simulink model "FiveStateAbsTcs"  (R2023b)
settings: configuration reference "VehicleFixed1ms" (kept outside this file)
undefined symbols (not defined in the file): CtrlBcuTrlrBrkGain, DiscIntNeverNeededParam, PlntWhlLdRadius
libraries: simulink x2
settings Model: DataDictionary=VirtualVehicleTemplate.sldd  ModifiedByFormat=The MathWorks, Inc.  Creator=The MathWorks, Inc.  LastModifiedBy=The MathWorks, Inc.
settings ConfigSetRef: SourceName=VehicleFixed1ms

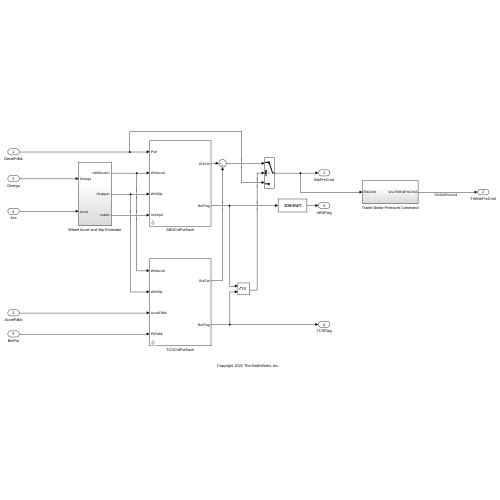
[thumbnail: Simulink's stored preview of the top-level diagram]
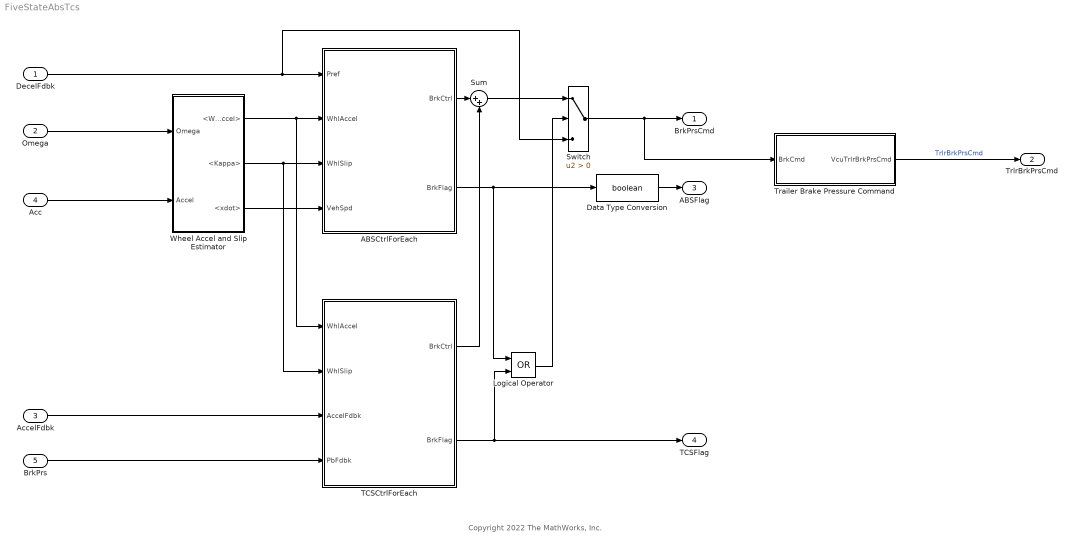
== system FiveStateAbsTcs ==
  note: Copyright 2022 The MathWorks, Inc.
  DecelFdbk : Inport  OutDataTypeStr=double  PortDimensions=1
  Omega : Inport  Port=2  OutDataTypeStr=double  PortDimensions=4
  AccelFdbk : Inport  Port=3  OutDataTypeStr=double  PortDimensions=1
  Acc : Inport  Port=4  OutDataTypeStr=double  PortDimensions=1
  BrkPrs : Inport  Port=5  OutDataTypeStr=double  PortDimensions=4
  ABSCtrlForEach : Subsystem  mask(Five-State ABS Control){Re=PlntWhlLdRadius, KappaOpt=-0.12, WhlAccelOpt=[-9.8,-9.8,-20,-20], v1=0, v5=0.55, v4=1, a2=-1.5, b=-1.5, A=4.5, a1=3.6, aMode=2}
      mask prompts: Re "Wheel effective radius, Re [m]:"; KappaOpt "Desired wheel slip ratio, KappaOpt [-]:"; WhlAccelOpt "Desired wheel acceleration, WhlAccelOpt [m/s^2]:"; v1 "Braking realease command, v1 [-]:"; v5 "Braking hold command, v5 [-]:"; v4 "Braking add command, v4 [-]:"; a2 "Threshold of State 1, a2 [m/s^2]:"; b "Threshold of State 2, b [m/s^2]:"; A "Threshold of State 3 and 4, A [m/s^2]:"; a1 "Threshold of State 5, a1 [m/s^2]:"
      mask help: This block determines brake pressure varying rate for each wheel once the ABS controller is activated. During ABS control, only wheel speed is directly regulated.
      mask init:
      | [~]=vehdynicon('vehdynblk',gcb);
      mask DialogControl vehParamGroup Prompt: Vehicle Parameter
      mask DialogControl ParameterGroupVar Prompt: Desired Control Parameters
      mask DialogControl Container3 Prompt: Braking Pressure Rates
      mask DialogControl Container4 Prompt: Wheel Acceleration Thresholds
  Data Type Conversion : DataTypeConversion  OutDataTypeStr=boolean  SaturateOnIntegerOverflow=off  RndMeth=Floor
  Logical Operator : Logic  Operator=OR  AllPortsSameDT=off  OutDataTypeStr=boolean
  Sum : Sum  Inputs=|++
  Switch : Switch  Criteria=u2 > Threshold  SaturateOnIntegerOverflow=off  InputSameDT=off
  TCSCtrlForEach : Subsystem  mask(Five-State TCS Control){Re=PlntWhlLdRadius, KappaOpt=0.12, WhlAccelOpt=[11, 11, 11, 11], v1=1.5, v5=-0.5, v4=-1.2, a2=-6, b=-10, A=-11, a1=-9, aMode=2}
      mask prompts: Re "Wheel effective radius, Re [m]:"; KappaOpt "Desired wheel slip ratio, KappaOpt [-]:"; WhlAccelOpt "Desired wheel acceleration, WhlAccelOpt [m/s^2]:"; v1 "Braking pressure rising rate, v1 [-]:"; v5 "Secondary braking pressure declining rate, v5 [-]:"; v4 "Braking pressure declining rate, v4 [-]:"; a2 "Threshold of State 1, a2 [m/s^2]:"; b "Threshold of State 2, b [m/s^2]:"; A "Threshold of State 3 and 4, A [m/s^2]:"; a1 "Threshold of State 5, a1 [m/s^2]:"
      mask help: This block determines brake pressure varying rate for each wheel once the TCS controller is activated. During TCS control, only wheel speed is directly regulated.
      mask init:
      | [~]=vehdynicon('vehdynblk',gcb);
      mask DialogControl vehParamGroup Prompt: Vehicle Parameter
      mask DialogControl ParameterGroupVar Prompt: Desired Control Parameters
      mask DialogControl Container3 Prompt: Braking Pressure Rates
      mask DialogControl Container4 Prompt: Wheel Acceleration Thresholds
  Trailer Brake Pressure Command : Subsystem
  Wheel Accel and Slip Estimator : Subsystem
  BrkPrsCmd : Outport  OutDataTypeStr=double  PortDimensions=4
  TrlrBrkPrsCmd : Outport  Port=2  PortDimensions=6  VectorParamsAs1DForOutWhenUnconnected=off
  ABSFlag : Outport  Port=3  OutDataTypeStr=boolean  PortDimensions=4
  TCSFlag : Outport  Port=4  OutDataTypeStr=double  PortDimensions=4
  wires:
  DecelFdbk/1 -> Switch/3, ABSCtrlForEach/1(Pref)
  Wheel Accel and Slip Estimator/3(<xdot>) -> ABSCtrlForEach/4(VehSpd)
  ABSCtrlForEach/1(BrkCtrl) -> Sum/1
  Sum/1 -> Switch/1
  BrkPrs/1 -> TCSCtrlForEach/4(PbFdbk)
  TCSCtrlForEach/1(BrkCtrl) -> Sum/2
  Logical Operator/1 -> Switch/2
  AccelFdbk/1 -> TCSCtrlForEach/3(AccelFdbk)
  Wheel Accel and Slip Estimator/1(<WhlAccel>) -> TCSCtrlForEach/1(WhlAccel), ABSCtrlForEach/2(WhlAccel)
  TCSCtrlForEach/2(BrkFlag) -> TCSFlag/1, Logical Operator/2
  ABSCtrlForEach/2(BrkFlag) -> Data Type Conversion/1, Logical Operator/1
  Wheel Accel and Slip Estimator/2(<Kappa>) -> TCSCtrlForEach/2(WhlSlip), ABSCtrlForEach/3(WhlSlip)
  Switch/1 -> Trailer Brake Pressure Command/1(BrkCmd), BrkPrsCmd/1
  Omega/1 -> Wheel Accel and Slip Estimator/1(Omega)
  Acc/1 -> Wheel Accel and Slip Estimator/2(Accel)
  Data Type Conversion/1 -> ABSFlag/1
  Trailer Brake Pressure Command/1(VcuTrlrBrkPrsCmd) -> TrlrBrkPrsCmd/1  "TrlrBrkPrsCmd"

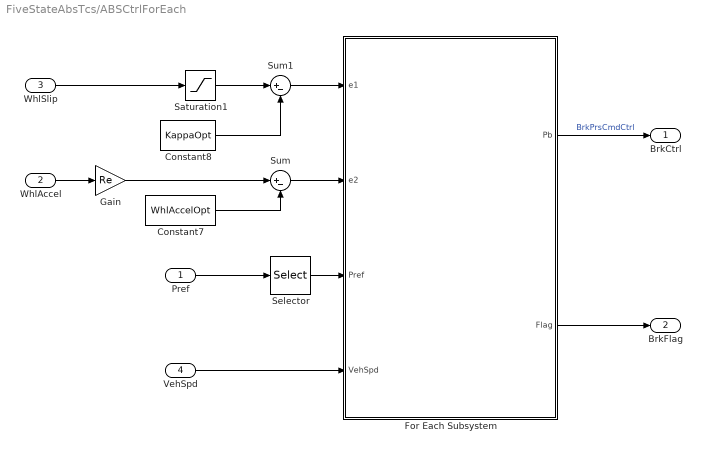
== system FiveStateAbsTcs/ABSCtrlForEach ==
  Pref : Inport
  WhlAccel : Inport  Port=2
  WhlSlip : Inport  Port=3
  VehSpd : Inport  Port=4
  Constant7 : Constant  Value=WhlAccelOpt
  Constant8 : Constant  Value=KappaOpt
  For Each Subsystem : Subsystem  TreatAsAtomicUnit=on
  Gain : Gain  Gain=Re
  Saturation1 : Saturate  UpperLimit=1  LowerLimit=-1
  Selector : Selector  InputPortWidth=1  IndexOptions=Index vector (dialog)  Indices=[1 1 1 1]  OutputSizes=1
  Sum : Sum  Inputs=|+-
  Sum1 : Sum  Inputs=|+-
  BrkCtrl : Outport
  BrkFlag : Outport  Port=2
  wires:
  Gain/1 -> Sum/1
  Constant8/1 -> Sum1/2
  WhlSlip/1 -> Saturation1/1
  Constant7/1 -> Sum/2
  Sum1/1 -> For Each Subsystem/1(e1)
  WhlAccel/1 -> Gain/1
  Saturation1/1 -> Sum1/1
  For Each Subsystem/2(Flag) -> BrkFlag/1
  Pref/1 -> Selector/1
  VehSpd/1 -> For Each Subsystem/4(VehSpd)
  For Each Subsystem/1(Pb) -> BrkCtrl/1  "BrkPrsCmdCtrl"
  Selector/1 -> For Each Subsystem/3(Pref)
  Sum/1 -> For Each Subsystem/2(e2)

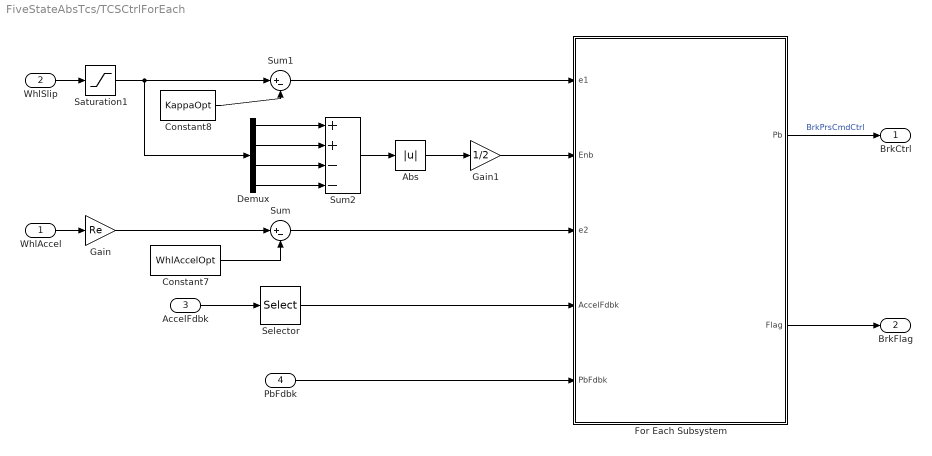
== system FiveStateAbsTcs/TCSCtrlForEach ==
  WhlAccel : Inport
  WhlSlip : Inport  Port=2
  AccelFdbk : Inport  Port=3
  PbFdbk : Inport  Port=4
  Abs : Abs  SaturateOnIntegerOverflow=off
  Constant7 : Constant  Value=WhlAccelOpt
  Constant8 : Constant  Value=KappaOpt
  Demux : Demux
  For Each Subsystem : Subsystem  TreatAsAtomicUnit=on
  Gain : Gain  Gain=Re
  Gain1 : Gain  Gain=1/2
  Saturation1 : Saturate  UpperLimit=1  LowerLimit=-1
  Selector : Selector  InputPortWidth=1  IndexOptions=Index vector (dialog)  Indices=[1 1 1 1]  OutputSizes=1
  Sum : Sum  Inputs=|+-
  Sum1 : Sum  Inputs=|+-
  Sum2 : Sum  Inputs=++--
  BrkCtrl : Outport
  BrkFlag : Outport  Port=2
  wires:
  Gain/1 -> Sum/1
  Constant8/1 -> Sum1/2
  WhlSlip/1 -> Saturation1/1
  Constant7/1 -> Sum/2
  Sum1/1 -> For Each Subsystem/1(e1)
  WhlAccel/1 -> Gain/1
  Saturation1/1 -> Demux/1, Sum1/1
  For Each Subsystem/2(Flag) -> BrkFlag/1
  AccelFdbk/1 -> Selector/1
  For Each Subsystem/1(Pb) -> BrkCtrl/1  "BrkPrsCmdCtrl"
  Selector/1 -> For Each Subsystem/4(AccelFdbk)
  Sum/1 -> For Each Subsystem/3(e2)
  PbFdbk/1 -> For Each Subsystem/5(PbFdbk)
  Demux/1 -> Sum2/1
  Demux/2 -> Sum2/2
  Demux/3 -> Sum2/3
  Demux/4 -> Sum2/4
  Sum2/1 -> Abs/1
  Abs/1 -> Gain1/1
  Gain1/1 -> For Each Subsystem/2(Enb)

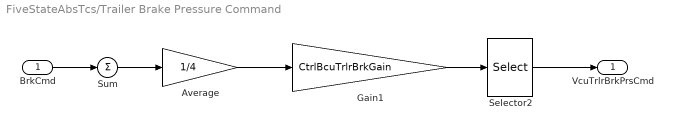
== system FiveStateAbsTcs/Trailer Brake Pressure Command ==
  BrkCmd : Inport
  Average : Gain  Gain=1/4
  Gain1 : Gain  Gain=CtrlBcuTrlrBrkGain
  Selector2 : Selector  InputPortWidth=1  IndexOptions=Index vector (dialog)  Indices=[1 1 1 1 1 1]  OutputSizes=1
  Sum : Sum  Inputs=+
  VcuTrlrBrkPrsCmd : Outport
  wires:
  Gain1/1 -> Selector2/1
  Average/1 -> Gain1/1
  BrkCmd/1 -> Sum/1
  Sum/1 -> Average/1
  Selector2/1 -> VcuTrlrBrkPrsCmd/1

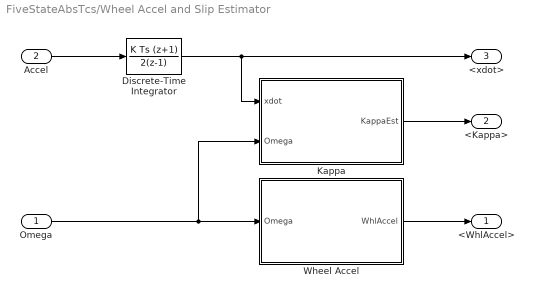
== system FiveStateAbsTcs/Wheel Accel and Slip Estimator ==
  Omega : Inport
  Accel : Inport  Port=2
  Discrete-Time Integrator : DiscreteIntegrator  IntegratorMethod=Integration: Trapezoidal  SampleTime=-1  ICPrevOutput=DiscIntNeverNeededParam  ICPrevScaledInput=DiscIntNeverNeededParam
  Kappa : Subsystem  TreatAsAtomicUnit=on
  Wheel Accel : Subsystem  TreatAsAtomicUnit=on
  <WhlAccel> : Outport
  <Kappa> : Outport  Port=2
  <xdot> : Outport  Port=3
  wires:
  Discrete-Time Integrator/1 -> <xdot>/1, Kappa/1(xdot)
  Accel/1 -> Discrete-Time Integrator/1
  Omega/1 -> Kappa/2(Omega), Wheel Accel/1(Omega)
  Wheel Accel/1(WhlAccel) -> <WhlAccel>/1
  Kappa/1(KappaEst) -> <Kappa>/1

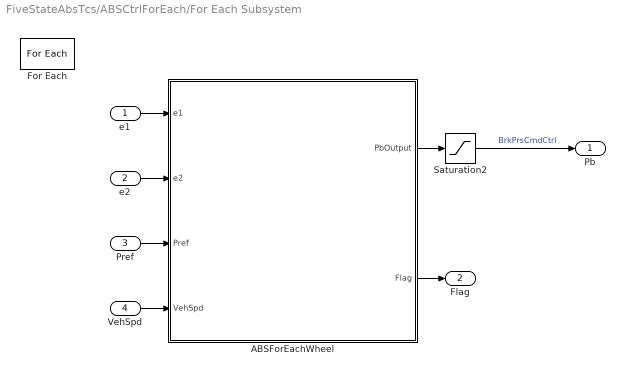
== system FiveStateAbsTcs/ABSCtrlForEach/For Each Subsystem ==
  e1 : Inport  Partition=on  PartitionDimension=1  PartitionWidth=1  PartitionOffset=0
  e2 : Inport  Port=2  Partition=on  PartitionDimension=1  PartitionWidth=1  PartitionOffset=0
  Pref : Inport  Port=3  Partition=on  PartitionDimension=1  PartitionWidth=1  PartitionOffset=0
  VehSpd : Inport  Port=4
  ABSForEachWheel : Stateflow chart  InitFcn=[~]=vehdynicon('vehdynblk',gcb);  TreatAsAtomicUnit=on
  For Each : ForEach  DisableCoverage=on
  Saturation2 : Saturate  UpperLimit=1  LowerLimit=0  ZeroCross=off
  Pb : Outport  ConcatenationDimension=1
  Flag : Outport  Port=2  ConcatenationDimension=1
  wires:
  e1/1 -> ABSForEachWheel/1(e1)
  e2/1 -> ABSForEachWheel/2(e2)
  VehSpd/1 -> ABSForEachWheel/4(VehSpd)
  Saturation2/1 -> Pb/1  "BrkPrsCmdCtrl"
  ABSForEachWheel/2(Flag) -> Flag/1
  ABSForEachWheel/1(PbOutput) -> Saturation2/1
  Pref/1 -> ABSForEachWheel/3(Pref)

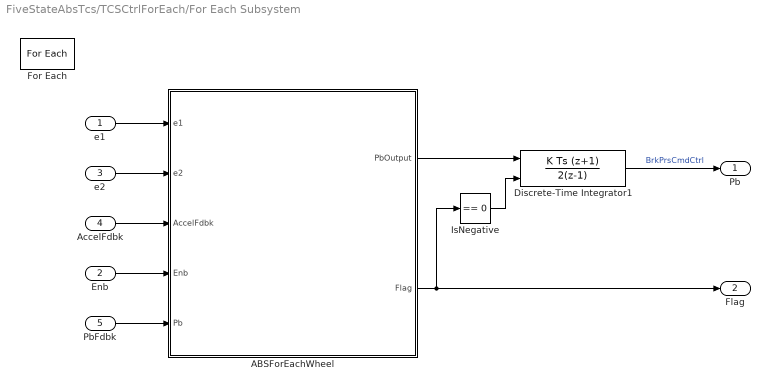
== system FiveStateAbsTcs/TCSCtrlForEach/For Each Subsystem ==
  e1 : Inport  Partition=on  PartitionDimension=1  PartitionWidth=1  PartitionOffset=0
  Enb : Inport  Port=2
  e2 : Inport  Port=3  Partition=on  PartitionDimension=1  PartitionWidth=1  PartitionOffset=0
  AccelFdbk : Inport  Port=4  Partition=on  PartitionDimension=1  PartitionWidth=1  PartitionOffset=0
  PbFdbk : Inport  Port=5  Partition=on  PartitionDimension=1  PartitionWidth=1  PartitionOffset=0
  ABSForEachWheel : Stateflow chart  InitFcn=[~]=vehdynicon('vehdynblk',gcb);  TreatAsAtomicUnit=on
  Discrete-Time Integrator1 : DiscreteIntegrator  IntegratorMethod=Integration: Trapezoidal  ExternalReset=rising  SampleTime=-1  LimitOutput=on  UpperSaturationLimit=1  LowerSaturationLimit=0  ICPrevOutput=DiscIntNeverNeededParam  ICPrevScaledInput=DiscIntNeverNeededParam
  For Each : ForEach  DisableCoverage=on
  IsNegative : simulink/Logic and Bit Operations/Compare To Zero  relop===  OutDataTypeStr=boolean  ZeroCross=off
  Pb : Outport  ConcatenationDimension=1
  Flag : Outport  Port=2  ConcatenationDimension=1
  wires:
  e1/1 -> ABSForEachWheel/1(e1)
  e2/1 -> ABSForEachWheel/2(e2)
  Discrete-Time Integrator1/1 -> Pb/1  "BrkPrsCmdCtrl"
  ABSForEachWheel/2(Flag) -> IsNegative/1, Flag/1
  ABSForEachWheel/1(PbOutput) -> Discrete-Time Integrator1/1
  AccelFdbk/1 -> ABSForEachWheel/3(AccelFdbk)
  Enb/1 -> ABSForEachWheel/4(Enb)
  PbFdbk/1 -> ABSForEachWheel/5(Pb)
  IsNegative/1 -> Discrete-Time Integrator1/2

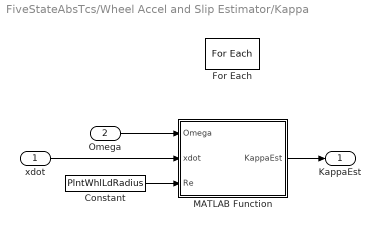
== system FiveStateAbsTcs/Wheel Accel and Slip Estimator/Kappa ==
  xdot : Inport
  Omega : Inport  Port=2  PortDimensions=1  Partition=on  PartitionDimension=1  PartitionWidth=1  PartitionOffset=0
  Constant : Constant  Value=PlntWhlLdRadius
  For Each : ForEach  DisableCoverage=on
  MATLAB Function : MATLAB Function  TreatAsAtomicUnit=on
  KappaEst : Outport  ConcatenationDimension=1
  wires:
  MATLAB Function/1(KappaEst) -> KappaEst/1
  xdot/1 -> MATLAB Function/2(xdot)
  Omega/1 -> MATLAB Function/1(Omega)
  Constant/1 -> MATLAB Function/3(Re)

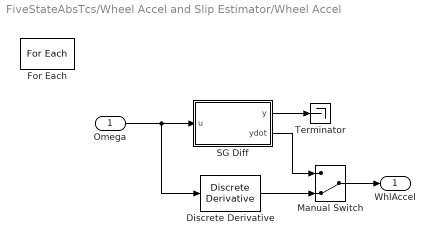
== system FiveStateAbsTcs/Wheel Accel and Slip Estimator/Wheel Accel ==
  Omega : Inport  PortDimensions=1  Partition=on  PartitionDimension=1  PartitionWidth=1  PartitionOffset=0
  Discrete Derivative : simulink/Discrete/Discrete Derivative  gainval=1.0  ICPrevScaledInput=0.0  OutMin=[]  OutMax=[]  OutDataType=fixdt(1, 16)  OutScaling=2^-10  DoSatur=off
  For Each : ForEach  DisableCoverage=on
  Manual Switch : ManualSwitch  CurrentSetting=0
  SG Diff : Subsystem  mask(Simplified Savitzky-Golay Differentiator){N=2, F=500, div0Tol=.001, aMode=2}
      mask prompts: N "Order, N [-]:"; F "Window,  F [-]:"; div0Tol "Ts div by 0 protection tolerance, [s]:"
      mask help:
      | Implements a Savitzky-Golay differentiator using double precision.
      | N is the polynomial to be fitted over window length F.
      mask init:
      | G=autosharedicon('autolibSGF',gcb);
  Terminator : Terminator
  WhlAccel : Outport  ConcatenationDimension=1
  wires:
  Omega/1 -> Discrete Derivative/1, SG Diff/1(u)
  SG Diff/1(y) -> Terminator/1
  Manual Switch/1 -> WhlAccel/1
  Discrete Derivative/1 -> Manual Switch/2
  SG Diff/2(ydot) -> Manual Switch/1

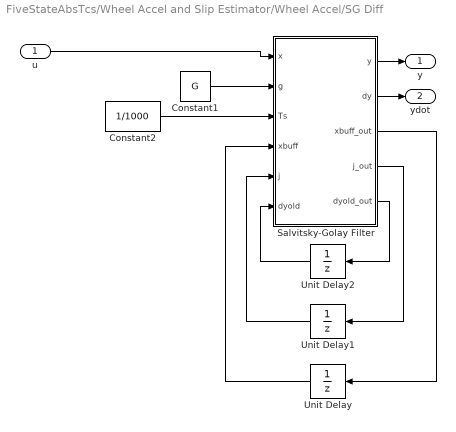
== system FiveStateAbsTcs/Wheel Accel and Slip Estimator/Wheel Accel/SG Diff ==
  u : Inport
  Constant1 : Constant  Value=G
  Constant2 : Constant  Value=1/1000
  Salvitsky-Golay Filter : MATLAB Function  TreatAsAtomicUnit=on
  Unit Delay : UnitDelay  SampleTime=-1  HasFrameUpgradeWarning=on
  Unit Delay1 : UnitDelay  SampleTime=-1  HasFrameUpgradeWarning=on
  Unit Delay2 : UnitDelay  SampleTime=-1  HasFrameUpgradeWarning=on
  y : Outport  VectorParamsAs1DForOutWhenUnconnected=off
  ydot : Outport  Port=2  VectorParamsAs1DForOutWhenUnconnected=off
  wires:
  Unit Delay/1 -> Salvitsky-Golay Filter/4(xbuff)
  Unit Delay1/1 -> Salvitsky-Golay Filter/5(j)
  Unit Delay2/1 -> Salvitsky-Golay Filter/6(dyold)
  Salvitsky-Golay Filter/3(xbuff_out) -> Unit Delay/1
  Salvitsky-Golay Filter/4(j_out) -> Unit Delay1/1
  Salvitsky-Golay Filter/5(dyold_out) -> Unit Delay2/1
  u/1 -> Salvitsky-Golay Filter/1(x)
  Constant1/1 -> Salvitsky-Golay Filter/2(g)
  Salvitsky-Golay Filter/2(dy) -> ydot/1
  Salvitsky-Golay Filter/1(y) -> y/1
  Constant2/1 -> Salvitsky-Golay Filter/3(Ts)

== stateflow chart FiveStateAbsTcs/TCSCtrlForEach/For Each Subsystem/ABSForEachWheel ==
  state TCSOff
    entry:
    PbOutput = 0;
    Flag = 0;
    during:
    PbOutput = 0;
  state Normal
    entry:
    PbOutput = 0;
    Flag = 0;
    during:
    PbOutput = 0;
  state TCSOn
    state Phase1
      entry:
      PbOutput = v1;
      Flag = 1;
    state Phase5
      entry:
      PbOutput = v5;
      Flag = 5;
    state Phase2
      entry:
      PbOutput = 0;
      Flag = 2;
    state Phase4
      entry:
      PbOutput = 0;
      Flag = 4;
    state Phase3
      entry:
      PbOutput = v4;
      Flag = 3;
    (default) -> Phase1
    Phase5 -> Phase1 : [e2 > a2]
    Phase1 -> Phase2 : [e2 <= b]
    Phase4 -> Phase5 : [e2 >= a1]
    Phase2 -> Phase3 : [e2 <= A]
    Phase3 -> Phase4 : [e2 > A]
  (default) -> TCSOff
  TCSOn -> TCSOff : [Pb <= 0 || AccelFdbk <= 0.2|| e1<0.1]
  Normal -> TCSOff [order 2] : [AccelFdbk <= 0]
  TCSOff -> Normal : [AccelFdbk > 0 && e2 > a2 && Enb > 0.3]
  Normal -> TCSOn [order 1] : [e1 > 0]
  data: e1 input; e2 input; PbOutput output; Flag output; b parameter; v1 parameter; v4 parameter; v5 parameter; A parameter; a2 parameter; a1 parameter; AccelFdbk input; Enb input; Pb input

== matlab function FiveStateAbsTcs/Wheel Accel and Slip Estimator/Kappa/MATLAB Function ==
  data: Omega input; xdot input; KappaEst output; Re input
function KappaEst = fcn(Omega, xdot, Re)

KappaEst = 0;
WhlSpd = Omega * Re;

if xdot*WhlSpd ~= 0
    KappaEst = (WhlSpd - xdot)/max([abs(xdot) abs(WhlSpd)]);
end

== matlab function FiveStateAbsTcs/Wheel Accel and Slip Estimator/Wheel Accel/SG Diff/Salvitsky-Golay Filter ==
  data: x input; y output; g input; dy output; Ts input; div0Tol parameter; xbuff input; j input int32; dyold input; xbuff_out output; j_out output int32; dyold_out output
function [y, dy, xbuff_out, j_out, dyold_out] = SGFilter(x,g,Ts,div0Tol, xbuff, j, dyold)%#codegen
%   Copyright 2016 The MathWorks, Inc.

coder.allowpcode('plain')
[y,dy, xbuff_out, j_out, dyold_out ] = autoblksSGFilter(x,g,Ts,div0Tol, xbuff, j, dyold);

== stateflow chart FiveStateAbsTcs/ABSCtrlForEach/For Each Subsystem/ABSForEachWheel ==
  state ABSOff
    entry:
    PbOutput = Pref;
    Flag = 0;
    during:
    PbOutput = Pref;
  state Normal
    entry:
    PbOutput = Pref;
    Flag = 0;
    during:
    PbOutput = Pref;
  state ABSOn
    state Phase1
      entry:
      PbOutput = v1;
      Flag = 1;
    state Phase5
      entry:
      PbOutput = v5;
      Flag = 5;
    state Phase2
      entry:
      PbOutput = 0;
      Flag = 2;
    state Phase4
      entry:
      PbOutput = 0;
      Flag = 4;
    state Phase3
      entry:
      PbOutput = v4;
      Flag = 3;
    (default) -> Phase1
    Phase5 -> Phase1 : [e2 < a2]
    Phase1 -> Phase2 : [e2 >= b]
    Phase4 -> Phase5 : [e2 <= a1]
    Phase2 -> Phase3 : [e2 >= A]
    Phase3 -> Phase4 : [e2 < A]
  (default) -> ABSOff
  ABSOn -> ABSOff : [abs(VehSpd) < 0.1 || Pref <= 0]
  Normal -> ABSOff [order 2] : [Pref <= 0]
  ABSOff -> Normal : [Pref > 0 && e2 < a2]
  Normal -> ABSOn [order 1] : [e1 < 0]
  data: e1 input; e2 input; PbOutput output; Flag output; b parameter; v1 parameter; v4 parameter; v5 parameter; A parameter; a2 parameter; a1 parameter; Pref input; VehSpd input
